simulink model "sampleModel1827"  (R2023a)
settings: Solver=VariableStepAuto  StartTime=0.0  StopTime=10.0  RelTol=1e-3
libraries: hdlsllib x7, simulink x2
settings Model: Creator=user1  LastModifiedBy=user1

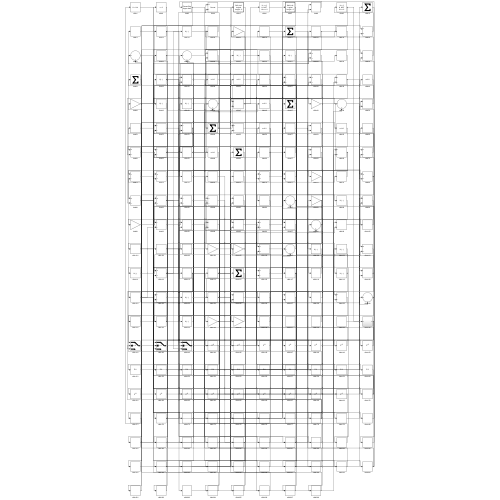
[thumbnail: Simulink's stored preview of the top-level diagram]
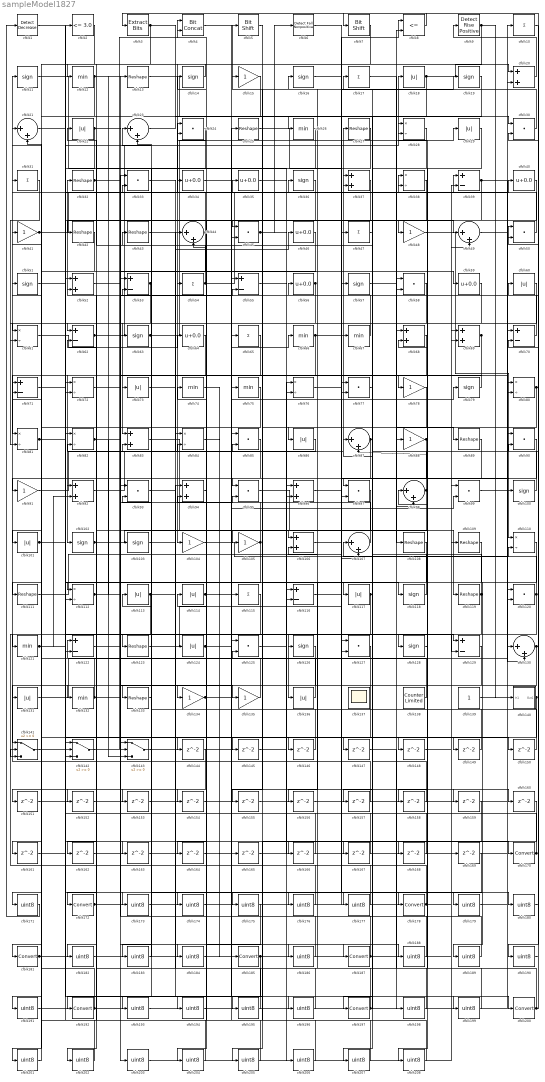
== system sampleModel1827 ==
  cfblk1 : simulink/Logic and Bit Operations/Detect Decrease  vinit=0.0  OutDataTypeStr=boolean
      settings: LibrarySourceBlock=|
      | hdlsllib/Logic and Bit
      | Operations/Detect
      | Decrease
  cfblk{10,17,31,47,54,65,115} (7 alike) : Sum  Inputs=+
  cfblk{11,14,16,19,36,51,57,63,79,100,102..103,118,126,128} (15 alike) : Signum
  cfblk{18,22,29,60,73,86,101,113..114,117,124,131,136} (13 alike) : Abs  SaturateOnIntegerOverflow=off
  cfblk{15,41,48,78,88,91,104..105,134..135} (10 alike) : Gain
  cfblk{20,37,52,68..69,83,92,94,96,106} (10 alike) : Sum
  cfblk{21,23,44,49,87,98,107,130} (8 alike) : Sum  Inputs=|++
  cfblk{13,25,27,32,42..43,89,108..109,111,119,123,133} (13 alike) : Reshape
  cfblk{28,38,61,72,76,80..82,84,110,112} (11 alike) : Product  Inputs=*/  RndMeth=Zero  SaturateOnIntegerOverflow=on
  cfblk{39,53,55,62,70..71,116,122,129} (9 alike) : Sum  Inputs=+-
  cfblk{12,26,66..67,74..75,121,132} (8 alike) : MinMax
  cfblk{24,30,33,45,50,58,77,85,90,93,95,97,99,120,125,127} (16 alike) : DotProduct  OutDataTypeStr=Inherit: Inherit via internal rule
  cfblk137 : Scope
      settings: Floating=on
  cfblk138 : hdlsllib/Sources/Counter Limited  uplimit=7  tsamp=-1
  cfblk139 : Constant  SampleTime=-1
  cfblk140 : Subsystem
      settings: LibrarySourceBlock=|
      | hdlsllib/Ports &
      | Subsystems/Subsystem
  cfblk141 : Switch  SaturateOnIntegerOverflow=off  InputSameDT=off
  cfblk142 : Switch  SaturateOnIntegerOverflow=off  InputSameDT=off
  cfblk143 : Switch  SaturateOnIntegerOverflow=off  InputSameDT=off
  cfblk{144..169} (26 alike) : Delay  SampleTime=1
  cfblk{170,172,178,181,185,187,192,197,200} (9 alike) : DataTypeConversion  SaturateOnIntegerOverflow=off  RndMeth=Floor
  cfblk{171,173..177,179..180,182..184,186,188..191,193..196,198..199,201..208} (30 alike) : DataTypeConversion  OutDataTypeStr=uint8  SaturateOnIntegerOverflow=off  RndMeth=Floor
  cfblk2 : hdlsllib/Logic and Bit Operations/Compare To Constant  relop=<=  const=3.0  OutDataTypeStr=boolean
  cfblk3 : simulink/Logic and Bit Operations/Extract Bits  bitsToExtract=Upper half  numBits=8  bitIdxRange=[0 7]  outScalingMode=Preserve fixed-point scaling
      settings: LibrarySourceBlock=|
      | hdlsllib/Logic and Bit
      | Operations/Extract Bits
  cfblk{34..35,40,46,56,59,64} (7 alike) : Bias  Bias=0.0  SaturateOnIntegerOverflow=off
  cfblk4 : hdlsllib/Logic and Bit Operations/Bit Concat  numInputs=2
  cfblk5 : hdlsllib/Logic and Bit Operations/Bit Shift  mode=Shift Left Logical  N=0
  cfblk6 : hdlsllib/Logic and Bit Operations/Detect Fall Nonpositive  vinit=0  OutDataTypeStr=boolean
  cfblk7 : hdlsllib/Logic and Bit Operations/Bit Shift  mode=Shift Left Logical  N=0
  cfblk8 : RelationalOperator  Operator=<=  OutDataTypeStr=boolean  InputSameDT=off
  cfblk9 : hdlsllib/Logic and Bit Operations/Detect Rise Positive  vinit=0  OutDataTypeStr=boolean
  wires:
  cfblk58/1 -> cfblk83/1
  cfblk84/1 -> cfblk115/1
  cfblk18/1 -> cfblk20/1, cfblk91/1
  cfblk79/1 -> cfblk78/1
  cfblk54/1 -> cfblk40/1, cfblk22/1, cfblk39/1
  cfblk142/1 -> cfblk4/1
  cfblk1/1 -> cfblk170/1
  cfblk92/1 -> cfblk27/1
  cfblk30/1 -> cfblk5/1
  cfblk129/1 -> cfblk11/1
  cfblk53/1 -> cfblk73/1, cfblk61/2
  cfblk41/1 -> cfblk36/1, cfblk48/1
  cfblk67/1 -> cfblk32/1
  cfblk11/1 -> cfblk116/1
  cfblk15/1 -> cfblk104/1
  cfblk117/1 -> cfblk167/1, cfblk201/1
  cfblk102/1 -> cfblk106/1, cfblk184/1
  cfblk120/1 -> cfblk107/1, cfblk136/1
  cfblk48/1 -> cfblk110/1
  cfblk63/1 -> cfblk29/1, cfblk46/1
  cfblk74/1 -> cfblk185/1
  cfblk93/1 -> cfblk187/1
  cfblk69/1 -> cfblk123/1, cfblk208/1
  cfblk64/1 -> cfblk102/1
  cfblk123/1 -> cfblk67/1
  cfblk32/1 -> cfblk143/1, cfblk58/2
  cfblk106/1 -> cfblk128/1
  cfblk45/1 -> cfblk6/1, cfblk149/1
  cfblk121/1 -> cfblk92/2, cfblk177/1, cfblk180/1
  cfblk87/1 -> cfblk97/1, cfblk117/1
  cfblk133/1 -> cfblk113/1
  cfblk127/1 -> cfblk172/1
  cfblk25/1 -> cfblk77/1
  cfblk20/1 -> cfblk9/1
  cfblk35/1 -> cfblk59/1
  cfblk130/1 -> cfblk7/1, cfblk164/1
  cfblk5/1 -> cfblk45/1
  cfblk36/1 -> cfblk45/2
  cfblk95/1 -> cfblk119/1
  cfblk96/1 -> cfblk19/1
  cfblk22/1 -> cfblk135/1, cfblk72/2
  cfblk140/1(Out1) -> cfblk161/1, cfblk162/1
  cfblk113/1 -> cfblk118/1, cfblk141/3, cfblk131/1, cfblk186/1
  cfblk82/1 -> cfblk55/2, cfblk143/3, cfblk188/1
  cfblk7/1 -> cfblk54/1
  cfblk62/1 -> cfblk18/1, cfblk80/2
  cfblk128/1 -> cfblk98/1
  cfblk44/1 -> cfblk24/1, cfblk71/1
  cfblk9/1 -> cfblk140/1(In1), cfblk182/1
  cfblk104/1 -> cfblk110/2
  cfblk78/1 -> cfblk86/1
  cfblk118/1 -> cfblk34/1
  cfblk119/1 -> cfblk28/2, cfblk156/1
  cfblk43/1 -> cfblk84/1
  cfblk46/1 -> cfblk62/1
  cfblk66/1 -> cfblk81/1, cfblk100/1
  cfblk132/1 -> cfblk53/1, cfblk41/1
  cfblk141/1 -> cfblk35/1
  cfblk13/1 -> cfblk55/1
  cfblk8/1 -> cfblk3/1
  cfblk50/1 -> cfblk24/2
  cfblk83/1 -> cfblk105/1
  cfblk17/1 -> cfblk89/1
  cfblk31/1 -> cfblk81/2
  cfblk107/1 -> cfblk14/1
  cfblk24/1 -> cfblk42/1
  cfblk114/1 -> cfblk99/2, cfblk165/1, cfblk176/1
  cfblk76/1 -> cfblk8/1
  cfblk136/1 -> cfblk122/1
  cfblk23/1 -> cfblk30/1
  cfblk42/1 -> cfblk111/1
  cfblk59/1 -> cfblk101/1
  cfblk88/1 -> cfblk87/2, cfblk151/1
  cfblk57/1 -> cfblk108/1
  cfblk65/1 -> cfblk192/1
  cfblk101/1 -> cfblk116/2, cfblk148/1
  cfblk49/1 -> cfblk120/1
  cfblk3/1 -> cfblk26/1, cfblk61/1
  cfblk14/1 -> cfblk12/1
  cfblk138/1 -> cfblk51/1
  cfblk143/1 -> cfblk96/2
  cfblk70/1 -> cfblk37/1
  cfblk81/1 -> cfblk28/1, cfblk129/2, cfblk168/1
  cfblk86/1 -> cfblk82/2
  cfblk91/1 -> cfblk44/1
  cfblk134/1 -> cfblk79/1, cfblk66/1
  cfblk85/1 -> cfblk92/1
  cfblk51/1 -> cfblk2/1
  cfblk75/1 -> cfblk181/1
  cfblk39/1 -> cfblk80/1, cfblk63/1
  cfblk111/1 -> cfblk57/1
  cfblk131/1 -> cfblk70/1
  cfblk105/1 -> cfblk122/2, cfblk44/2
  cfblk80/1 -> cfblk50/1, cfblk95/1
  cfblk26/1 -> cfblk132/1
  cfblk139/1 -> cfblk20/2
  cfblk89/1 -> cfblk133/1
  cfblk124/1 -> cfblk126/1, cfblk159/1
  cfblk103/1 -> cfblk129/1
  cfblk61/1 -> cfblk64/1
  cfblk12/1 -> cfblk142/3, cfblk144/1
  cfblk135/1 -> cfblk84/2
  cfblk56/1 -> cfblk76/2, cfblk191/1
  cfblk99/1 -> cfblk130/2
  cfblk100/1 -> cfblk43/1
  cfblk126/1 -> cfblk141/1
  cfblk90/1 -> cfblk178/1
  cfblk2/1 -> cfblk121/1
  cfblk77/1 -> cfblk17/1
  cfblk116/1 -> cfblk47/1
  cfblk98/1 -> cfblk134/1, cfblk31/1, cfblk38/2, cfblk112/1
  cfblk72/1 -> cfblk38/1
  cfblk68/1 -> cfblk197/1
  cfblk60/1 -> cfblk77/2
  cfblk34/1 -> cfblk49/1
  cfblk112/1 -> cfblk103/1, cfblk13/1, cfblk95/2
  cfblk21/1 -> cfblk200/1
  cfblk37/1 -> cfblk145/1
  cfblk145/1 -> cfblk76/1
  cfblk109/1 -> cfblk146/1
  cfblk146/1 -> cfblk85/2
  cfblk47/1 -> cfblk147/1
  cfblk148/1 -> cfblk49/2
  cfblk149/1 -> cfblk23/2
  cfblk6/1 -> cfblk150/1
  cfblk150/1 -> cfblk4/2
  cfblk151/1 -> cfblk8/2
  cfblk40/1 -> cfblk152/1
  cfblk152/1 -> cfblk130/1
  cfblk115/1 -> cfblk153/1
  cfblk153/1 -> cfblk107/2
  cfblk38/1 -> cfblk154/1
  cfblk154/1 -> cfblk98/2
  cfblk108/1 -> cfblk155/1
  cfblk155/1 -> cfblk50/2
  cfblk156/1 -> cfblk97/2
  cfblk28/1 -> cfblk157/1
  cfblk157/1 -> cfblk82/1
  cfblk29/1 -> cfblk158/1
  cfblk158/1 -> cfblk87/1
  cfblk55/1 -> cfblk160/1
  cfblk162/1 -> cfblk39/2
  cfblk71/1 -> cfblk163/1
  cfblk163/1 -> cfblk96/1
  cfblk164/1 -> cfblk69/2
  cfblk165/1 -> cfblk120/2
  cfblk122/1 -> cfblk166/1
  cfblk166/1 -> cfblk83/2
  cfblk167/1 -> cfblk142/1
  cfblk168/1 -> cfblk142/2
  cfblk170/1 -> cfblk58/1, cfblk56/1
  cfblk144/1 -> cfblk171/1
  cfblk171/1 -> cfblk1/1
  cfblk172/1 -> cfblk143/2, cfblk69/1
  cfblk161/1 -> cfblk173/1
  cfblk173/1 -> cfblk127/1
  cfblk97/1 -> cfblk174/1
  cfblk174/1 -> cfblk127/2
  cfblk33/1 -> cfblk175/1
  cfblk176/1 -> cfblk33/1
  cfblk177/1 -> cfblk33/2
  cfblk178/1 -> cfblk72/1, cfblk106/2, cfblk141/2
  cfblk16/1 -> cfblk179/1
  cfblk179/1 -> cfblk90/1
  cfblk180/1 -> cfblk90/2
  cfblk181/1 -> cfblk112/2, cfblk124/1
  cfblk182/1 -> cfblk75/1
  cfblk169/1 -> cfblk183/1
  cfblk183/1 -> cfblk53/2
  cfblk184/1 -> cfblk169/1
  cfblk185/1 -> cfblk15/1, cfblk202/1
  cfblk186/1 -> cfblk74/1
  cfblk187/1 -> cfblk88/1, cfblk23/1
  cfblk188/1 -> cfblk93/1
  cfblk110/1 -> cfblk189/1
  cfblk189/1 -> cfblk93/2
  cfblk10/1 -> cfblk190/1
  cfblk190/1 -> cfblk60/1
  cfblk191/1 -> cfblk10/1
  cfblk192/1 -> cfblk71/2, cfblk25/1
  cfblk27/1 -> cfblk193/1
  cfblk193/1 -> cfblk65/1
  cfblk94/1 -> cfblk194/1
  cfblk194/1 -> cfblk85/1
  cfblk160/1 -> cfblk195/1
  cfblk195/1 -> cfblk94/1
  cfblk73/1 -> cfblk196/1
  cfblk196/1 -> cfblk94/2
  cfblk197/1 -> cfblk16/1, cfblk109/1, cfblk37/2
  cfblk147/1 -> cfblk198/1
  cfblk198/1 -> cfblk68/1
  cfblk4/1 -> cfblk199/1
  cfblk199/1 -> cfblk68/2
  cfblk200/1 -> cfblk30/2, cfblk62/2, cfblk70/2
  cfblk201/1 -> cfblk21/1
  cfblk202/1 -> cfblk21/2
  cfblk52/1 -> cfblk203/1
  cfblk203/1 -> cfblk99/1
  cfblk175/1 -> cfblk204/1
  cfblk204/1 -> cfblk52/1
  cfblk159/1 -> cfblk205/1
  cfblk205/1 -> cfblk52/2
  cfblk125/1 -> cfblk206/1
  cfblk206/1 -> cfblk114/1
  cfblk19/1 -> cfblk207/1
  cfblk207/1 -> cfblk125/1
  cfblk208/1 -> cfblk125/2

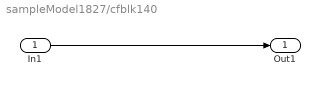
== system sampleModel1827/cfblk140 ==
  In1 : Inport
  Out1 : Outport
  wires:
  In1/1 -> Out1/1
